simulink model "tutorial6"  (Simulink 2.20)
settings: Solver=ode5  StartTime=0.0  StopTime=tstop  FixedStep=tstep  MaxStep=tstep  RelTol=1e-3  AbsTol=1e-3
values from neighbouring files (symbols this model uses):
  gf = 1    [tutorial6prep.m]
settings Model: SaveTime=off  SaveOutput=off  ConsistencyChecking=off  RTWPlaceOutputsASAP=off

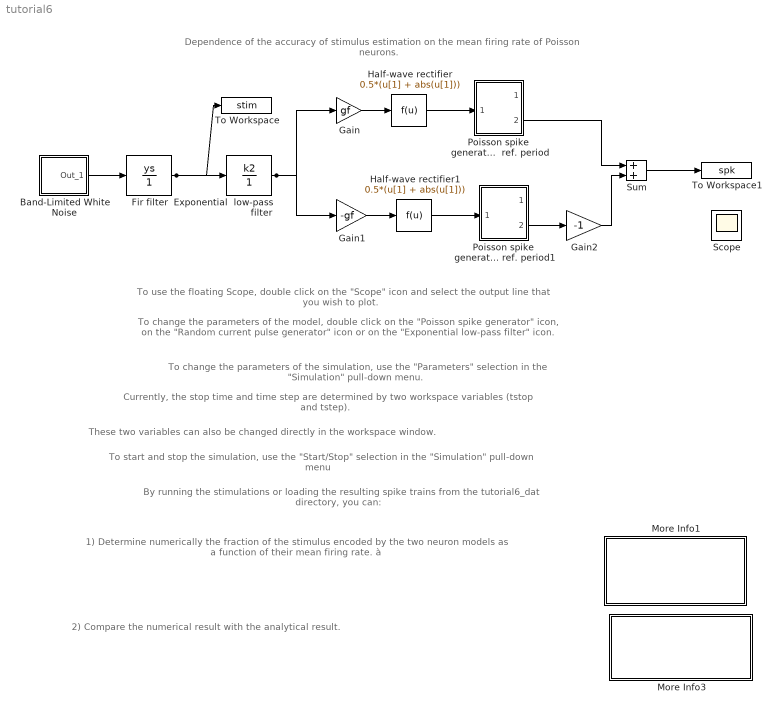
== system tutorial6 ==
  note: Dependence of the accuracy of stimulus estimation on the mean firing rate of Poisson neurons.
  note: To use the floating Scope, double click on the "Scope" icon and select the output line that you wish to plot.
  note: To change the parameters of the model, double click on the  "Poisson spike generator" icon, on the "Random
      | current pulse generator" icon or on the "Exponential low-pass filter" icon.
  note: To change the parameters of the simulation, use the "Parameters" selection in the "Simulation" pull-down menu.
  note: Currently, the stop time and time step are determined by two workspace variables (tstop and tstep).
  note: To start and stop the simulation, use the "Start/Stop" selection in the "Simulation" pull-down menu
  note: These two variables can also be changed directly in the workspace window.
  note: By running the stimulations or loading the resulting spike trains from the tutorial6_dat directory, you can:
  note: 1) Determine numerically the fraction of the stimulus encoded by the two neuron models
      | as a  function of  their mean firing rate.à
  note: 2) Compare the numerical result with the analytical result.
  Band-Limited White Noise : Subsystem  mask(Discrete time white noise. ){@1=tstep, @2=0.1, @3=[23341]}
      mask prompts: @1 "time step [msec]"; @2 "standard deviation [nA]"; @3 "random seed"
      mask help: Discrete time white noise
      mask init:
      | dt = @1; sigma = @2; seed = @3; r = rand(1,12); r2 = [r(1),r;r,r(12)]; t =[1:13;1:13];
      mask Help: Generates a sequence of normally distributed random numbers with standard deviation sigma
      mask Display: plot(t(:),r2(:))
  Exponential  low-pass filter : DiscreteFilter  Numerator=k2  Denominator=1  SampleTime=dt  mask(Exponential low-pass filter){@1=20, @2=1024, @3=tstep}
      mask prompts: @1 "Time constant [msec]"; @2 "Number of  points"; @3 "time step [msec]"
      mask help: Parameters
      mask init:
      | tau = @1; n = @2; dt = @3; t = [0:1:n-1]*dt; k2 = exp(-t/tau) ; k2 = k2/norm(k2);
      mask Display: plot(t,k2);
  Fir filter : DiscreteFilter  Numerator=ys  Denominator=1  SampleTime=dt  mask(Fir1 filter){@1=100, @2=1024, @3=tstep}
      mask prompts: @1 "Cut-off frequency [Hz]"; @2 "Number of  points"; @3 "time step [msec]"
      mask help: Parameters
      mask init:
      | fc = @1; n = @2; dt = @3; fn = 1/(2*dt*1e-3); ys = fir1(n,fc/fn); ys = ys/norm(ys);
      mask Display: plot((1:n+1),ys);
  Gain : Gain  Gain=gf
  Gain1 : Gain  Gain=-gf
  Gain2 : Gain  Gain=-1
  Half-wave rectifier : Fcn  Expr=0.5*(u[1] + abs(u[1]))  mask(half-wave rectifier){}
      mask init:
      | x = [-2:0.1:2]; y = 0.5*(x+abs(x));
      mask Display: plot(x,y);
  Half-wave rectifier1 : Fcn  Expr=0.5*(u[1] + abs(u[1]))  mask(half-wave rectifier){}
      mask init:
      | x = [-2:0.1:2]; y = 0.5*(x+abs(x));
      mask Display: plot(x,y);
  More Info1 : Subsystem
      mask Display: disp('Numerical estimation \nof the fraction of the \nstimulus encoded as \na function of mean \nfiring rate')
  More Info3 : Subsystem
      mask Display: disp('Comparison with the\n theoretical result')
  Poisson spike  generator with  ref. period : Subsystem  mask(I&F p. thres., ref. per.){@1=tstep, @2=10, @3=.5, @4=tstep}
      mask prompts: @1 "time step [msec]"; @2 "mean threshold [mV]"; @3 "Capacitance [nF]"; @4 "refractory period [msec]"
      mask help: Parameters
      mask init:
      | dt = @1; thres = @2; C = @3; ref = @4;
      mask Help: For a detailled description of the model, please type 'help piandfr' in the main matlab window
      mask Display: disp('Vm \n\n spikes')
  Poisson spike  generator with  ref. period1 : Subsystem  mask(I&F p. thres., ref. per.){@1=tstep, @2=10, @3=.5, @4=tstep}
      mask prompts: @1 "time step [msec]"; @2 "mean threshold [mV]"; @3 "Capacitance [nF]"; @4 "refractory period [msec]"
      mask help: Parameters
      mask init:
      | dt = @1; thres = @2; C = @3; ref = @4;
      mask Help: For a detailled description of the model, please type 'help piandfr' in the main matlab window
      mask Display: disp('Vm \n\n spikes')
  Scope : Scope
      settings: TickLabels=on  TimeRange=500.000000  YMin=-2.000000  YMax=2.000000  SaveToWorkspace=off  SaveName=ScopeData
  Sum : Sum  Inputs=++
  To Workspace : ToWorkspace  VariableName=stim  SampleTime=0
      settings: Buffer=ceil(tstop/tstep)
  To Workspace1 : ToWorkspace  VariableName=spk  SampleTime=0
      settings: Buffer=ceil(tstop/tstep)
  wires:
  Half-wave rectifier/1 -> Poisson spike  generator with  ref. period/1(in_1)
  Half-wave rectifier1/1 -> Poisson spike  generator with  ref. period1/1(in_1)
  Gain1/1 -> Half-wave rectifier1/1
  Gain/1 -> Half-wave rectifier/1
  Band-Limited White Noise/1(Out_1) -> Fir filter/1
  Poisson spike  generator with  ref. period1/2(out_1) -> Gain2/1
  Sum/1 -> To Workspace1/1
  Poisson spike  generator with  ref. period/2(out_1) -> Sum/1
  Fir filter/1 -> Exponential  low-pass filter/1, To Workspace/1
  Gain2/1 -> Sum/2
  Exponential  low-pass filter/1 -> Gain1/1, Gain/1

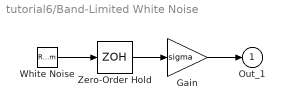
== system tutorial6/Band-Limited White Noise ==
  Gain : Gain  Gain=sigma
  White Noise : RandomNumber  Mean=0  Variance=1  Seed=seed  SampleTime=-1
  Zero-Order Hold : ZeroOrderHold  SampleTime=dt
  Out_1 : Outport  Port=1  InitialOutput=0
  wires:
  Zero-Order Hold/1 -> Gain/1
  Gain/1 -> Out_1/1
  White Noise/1 -> Zero-Order Hold/1

== system tutorial6/More Info1 ==
  note: To compute the accuracy of stimulus estimation
      | as a function of mean firing rate, you can:
  note: 1) Call the script "stestf1" which will sequentially
      | load in the workspace the results of simulations of the
      | model for different values of the gain gf.
  note: These results are stored in the directory "tutorial6_dat".
      | From the results (spike trains and stimuli) the script will
      | compute the mean firing rate and coding fraction and
      | plot them.
  note: 2) Perform the actual simulations by calling the script
      | "stestf" (this is a computationally very intensive simulation).
      | The first time that "stestf" is called, it will ask for:
  note: -a vector of values for gf (answer: [0.25:0.25:2]).
  note: -the name of the variable to be changed for each new
      | simulation (answer: gf).
  note: -the name of the variable containing the spike trains
      | (answer: spk).
  note: -the name of the variable containing the stimulus
      | (answer: stim).
  note: -the name of the model (answer: tutorial6).
  note: For subsequent calls, stestf will use the same values for
      | the variables as entered in the previous steps.

== system tutorial6/More Info3 ==
  note: To compare the  numerical results with the analytical formula,
      | enter:
  note: hold on
  note: stesttheor(0.1,100,20,10,100,10)
  note: in the main matlab window. The parameters are:
  note: 0.1 = standard deviation of the stimulus (in nA).
  note: 100 = cut-off frequency of the stimulus (in Hz).
  note: 20 = time constant of low-pass filtering (in msec).
  note: 10 = minimum firing frequency of each neuron (in Hz).
  note: 100 = maximal firing frequency of each neuron (in Hz).
  note: 10 = increment step in firing frequency (in Hz).

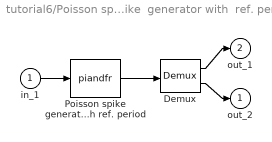
== system tutorial6/Poisson spike  generator with  ref. period ==
  in_1 : Inport  Port=1  PortWidth=-1  SampleTime=-1
  Demux : Demux  Outputs=2
  Poisson spike generator with ref. period : S-Function  FunctionName=piandfr  Parameters=dt,thres,C, ref  PortCounts=[]  SFunctionModules=''
  out_2 : Outport  Port=1  InitialOutput=0
  out_1 : Outport  Port=2  InitialOutput=0
  wires:
  Poisson spike generator with ref. period/1 -> Demux/1
  Demux/1 -> out_1/1
  Demux/2 -> out_2/1
  in_1/1 -> Poisson spike generator with ref. period/1

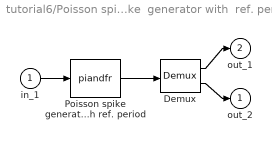
== system tutorial6/Poisson spike  generator with  ref. period1 ==
  in_1 : Inport  Port=1  PortWidth=-1  SampleTime=-1
  Demux : Demux  Outputs=2
  Poisson spike generator with ref. period : S-Function  FunctionName=piandfr  Parameters=dt,thres,C, ref  PortCounts=[]  SFunctionModules=''
  out_2 : Outport  Port=1  InitialOutput=0
  out_1 : Outport  Port=2  InitialOutput=0
  wires:
  Poisson spike generator with ref. period/1 -> Demux/1
  Demux/1 -> out_1/1
  Demux/2 -> out_2/1
  in_1/1 -> Poisson spike generator with ref. period/1
